simulink model "cascaded_5_lvl"  (R2023a)
settings: Solver=ode4  StartTime=0.0  StopTime=0.1  FixedStep=1e-5  RelTol=1e-3  EnableMultiTasking=on
libraries: spsIGBTDiodeLib x24, simulink x12, spsDCVoltageSourceLib x6, spsSeriesRLCBranchLib x3, spsGroundLib x2, spsThreePhaseVIMeasurementLib x1, spspowerguiLib x1
settings Model: Creator=Rini Roni  LastModifiedBy=dhana
settings SolverCC: AlgebraicLoopSolver=TrustRegion
settings DataIOCC: LimitDataPoints=on  SaveFormat=Array  ReturnWorkspaceOutputs=off
settings OptimizationCC: LifeSpan=inf
settings DebuggingCC: UnderspecifiedInitializationDetection=Classic  MergeDetectMultiDrivingBlocksExec=none  SolverPrmCheckMsg=warning  UnconnectedInputMsg=warning  UnconnectedOutputMsg=warning  UnconnectedLineMsg=warning  StateNameClashWarn=warning  SFUnexpectedBacktrackingDiag=warning  SFNoUnconditionalDefaultTransitionDiag=warning  SFExecutionAtInitializationDiag=none  ArithmeticOperatorsInVariantConditions=warning
settings HardwareCC: ProdBitPerPointer=32  ProdBitPerSizeT=32  ProdBitPerPtrDiffT=32  ProdLargestAtomicFloat=None  ProdIntDivRoundTo=Undefined  ProdEndianess=Unspecified  ProdWordSize=32  ProdHWDeviceType=32-bit Generic
settings ModelReferenceCC: EnableRefExpFcnMdlSchedulingChecks=on  PropagateSignalLabelsOutOfModel=off
settings SFSimCC: SimUseLocalCustomCode=off  CustomCodeUndefinedFunction=UseInterfaceOnly
settings RTWCC: RTWUseLocalCustomCode=off
settings CodeAppCC: StateflowObjectComments=on
settings GRTTargetCC: TargetLangStandard=C89/C90 (ANSI)
settings ConfigComp: CovMetricSettings=dw  CovSaveCumulativeToWorkspaceVar=on  CovSaveSingleToWorkspaceVar=on  CovExternalEMLEnable=off
settings SimscapeCC: SimscapeNormalizeSystem=off

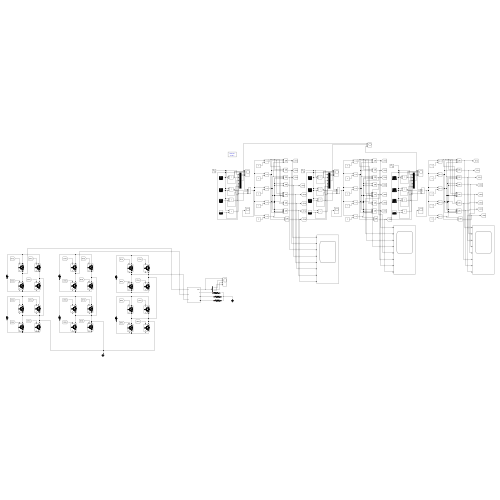
[thumbnail: Simulink's stored preview of the top-level diagram]
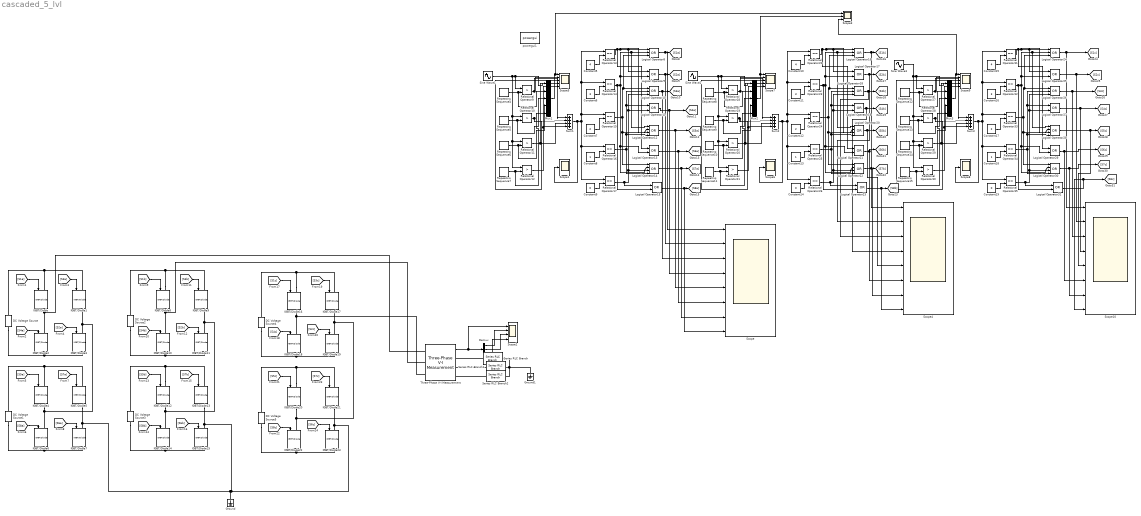
== system cascaded_5_lvl ==
  Constant10 : Constant  Value=4
  Constant11 : Constant  Value=3
  Constant12 : Constant  Value=2
  Constant13 : Constant
  Constant14 : Constant  Value=0
  Constant15 : Constant  Value=4
  Constant16 : Constant  Value=3
  Constant17 : Constant  Value=2
  Constant18 : Constant
  Constant19 : Constant  Value=0
  Constant5 : Constant  Value=4
  Constant6 : Constant  Value=3
  Constant7 : Constant  Value=2
  Constant8 : Constant
  Constant9 : Constant  Value=0
  DC Voltage Source{,1..5} (6 alike) : spsDCVoltageSourceLib/DC Voltage Source  Amplitude=50  Measurements=None
  Demux : Demux  Outputs=3
  Ground : spsGroundLib/Ground  LConnTagsString=a
  Ground1 : spsGroundLib/Ground  LConnTagsString=a
  IGBT/Diode{,1..23} (24 alike) : spsIGBTDiodeLib/IGBT//Diode  Ron=1e-3  Rs=1e5  Cs=inf  Measurements=on
  Logical Operator{8,10,16,18,24,26} (6 alike) : Logic  Operator=OR  Inputs=3  AllPortsSameDT=off  OutDataTypeStr=boolean
  Logical Operator{9,11,13,15,17,19,21,23,25,27,29,31} (12 alike) : Logic  Operator=OR  AllPortsSameDT=off  OutDataTypeStr=boolean
  Logical Operator{12,14,20,22,28,30} (6 alike) : Logic  Operator=OR  Inputs=4  AllPortsSameDT=off  OutDataTypeStr=boolean
  Mux1 : Mux  Inputs=5
  Mux2 : Mux  Inputs=5
  Mux3 : Mux  Inputs=5
  Relational Operator{9..12,18..21,27..30} (12 alike) : RelationalOperator  Operator=>  OutDataTypeStr=boolean  InputSameDT=off
  Relational Operator{13..17,22..26,31..35} (15 alike) : RelationalOperator  Operator===  OutDataTypeStr=boolean  InputSameDT=off
  Repeating Sequence10 : simulink/Sources/Repeating Sequence  rep_seq_t=[0 1 2 ]*[1/5000]  rep_seq_y=[-1 0 -1]
  Repeating Sequence11 : simulink/Sources/Repeating Sequence  rep_seq_t=[0 1 2 ]*[1/5000]  rep_seq_y="[-2  -1 -2]"
  Repeating Sequence12 : simulink/Sources/Repeating Sequence  rep_seq_t=[0 1 2 ]*[1/5000]  rep_seq_y=[1 2 1]
  Repeating Sequence13 : simulink/Sources/Repeating Sequence  rep_seq_t=[0 1 2 ]*[1/5000]  rep_seq_y=[0 1 0]
  Repeating Sequence14 : simulink/Sources/Repeating Sequence  rep_seq_t=[0 1 2 ]*[1/5000]  rep_seq_y=[-1 0 -1]
  Repeating Sequence15 : simulink/Sources/Repeating Sequence  rep_seq_t=[0 1 2 ]*[1/5000]  rep_seq_y="[-2  -1 -2]"
  Repeating Sequence4 : simulink/Sources/Repeating Sequence  rep_seq_t=[0 1 2 ]*[1/5000]  rep_seq_y=[1 2 1]
  Repeating Sequence5 : simulink/Sources/Repeating Sequence  rep_seq_t=[0 1 2 ]*[1/5000]  rep_seq_y=[0 1 0]
  Repeating Sequence6 : simulink/Sources/Repeating Sequence  rep_seq_t=[0 1 2 ]*[1/5000]  rep_seq_y=[-1 0 -1]
  Repeating Sequence7 : simulink/Sources/Repeating Sequence  rep_seq_t=[0 1 2 ]*[1/5000]  rep_seq_y="[-2  -1 -2]"
  Repeating Sequence8 : simulink/Sources/Repeating Sequence  rep_seq_t=[0 1 2 ]*[1/5000]  rep_seq_y=[1 2 1]
  Repeating Sequence9 : simulink/Sources/Repeating Sequence  rep_seq_t=[0 1 2 ]*[1/5000]  rep_seq_y=[0 1 0]
  Scope : Scope  NumInputPorts=8
  Scope1 : Scope
  Scope10 : Scope  NumInputPorts=8
  Scope2 : Scope  NumInputPorts=4
  Scope3 : Scope  NumInputPorts=3
  Scope4 : Scope  NumInputPorts=8
  Scope5 : Scope  NumInputPorts=5
  Scope6 : Scope
  Scope7 : Scope  NumInputPorts=5
  Scope8 : Scope
  Scope9 : Scope  NumInputPorts=5
  Series RLC Branch : spsSeriesRLCBranchLib/Series RLC Branch  LConnTagsString=__new0  RConnTagsString=__new0  BranchType=R  Resistance=500  Inductance=1e-3  SetiL0=off  InitialCurrent=0  Capacitance=1e-6  Setx0=off  InitialVoltage=0  Measurements=Branch voltage
  Series RLC Branch1 : spsSeriesRLCBranchLib/Series RLC Branch  LConnTagsString=__new0  RConnTagsString=__new0  BranchType=R  Resistance=100  Inductance=1e-3  SetiL0=off  InitialCurrent=0  Capacitance=1e-6  Setx0=off  InitialVoltage=0  Measurements=Branch voltage
  Series RLC Branch2 : spsSeriesRLCBranchLib/Series RLC Branch  LConnTagsString=__new0  RConnTagsString=__new0  BranchType=R  Resistance=250  Inductance=1e-3  SetiL0=off  InitialCurrent=0  Capacitance=1e-6  Setx0=off  InitialVoltage=0  Measurements=Branch voltage
  Sine Wave1 : Sin  Amplitude=2  Frequency=2*pi*50  SampleTime=0
  Sine Wave2 : Sin  Amplitude=2  Frequency=2*pi*50  Phase=4*pi/3  SampleTime=0
  Sine Wave3 : Sin  Amplitude=2  Frequency=2*pi*50  Phase=2*pi/3  SampleTime=0
  Sum1 : Sum  Inputs=|++++
  Sum2 : Sum  Inputs=|++++
  Sum3 : Sum  Inputs=|++++
  Three-Phase V-I Measurement : spsThreePhaseVIMeasurementLib/Three-Phase V-I Measurement  VoltageMeasurement=phase-to-ground  SetLabelV=off  LabelV=Vabc  Vpu=off  VpuLL=off  CurrentMeasurement=no  SetLabelI=off  LabelI=Iabc  Ipu=off  Pbase=100e6  Vbase=500e3  OutputType=Complex  PhasorSimulation=off  PSBequivalent=0
  powergui1 : spspowerguiLib/powergui  Priority=1  SimulationMode=Discrete  SampleTime=1e-5  frequency=60  Iterations=50  frequencyindice=0  Pbase=100e6  ErrMax=1e-4  UnitsV=kV  UnitsW=MW  buscounter=0  FunctionMessages=off  echomessages=off  EnableUseOfTLC=off  CurrentSourceSwitches=off  DisableSnubberDevices=off  DisableRonSwitches=off  DisableVfSwitches=off  DisplayEquations=off  AutomaticDiscreteSolvers=off  SolverType=Tustin  Interpol=off  ExternalGateDelay=off  methode=off  Ts=0  x0status=blocks  SPID=off  SwTol=0  HookPort=off  NonlinearTolerance=1e-4  nMaxIteration=100  ContinueOnMaxIteration=off  RestoreLinks=warning  ResistiveCurrentMeasurement=off  Frange=[0:2:500]  Ylog=off  Xlog=on  ShowGrid=off  save=off  variable=ZData  structure=ScopeData  ZoomFFT=off  StartTime=0.02  cycles=1  DisplayStyle=1  fundamental=50  FreqAxis=off  MaxFrequency=1000  frequencyindicesteady=1  RmsSteady=1  display=off
  wires:
  [S1a] -> IGBT/Diode/1
  [S4a] -> IGBT/Diode2/1
  [S3a] -> IGBT/Diode1/1
  [S2a] -> IGBT/Diode3/1
  [S5a] -> IGBT/Diode4/1
  [S8a] -> IGBT/Diode6/1
  [S7a] -> IGBT/Diode5/1
  [S6a] -> IGBT/Diode7/1
  [S1b] -> IGBT/Diode8/1
  [S6b] -> IGBT/Diode15/1
  [S7b] -> IGBT/Diode13/1
  [S8b] -> IGBT/Diode14/1
  [S2b] -> IGBT/Diode11/1
  [S3b] -> IGBT/Diode9/1
  [S4b] -> IGBT/Diode10/1
  [S5b] -> IGBT/Diode12/1
  [S1c] -> IGBT/Diode16/1
  [S6c] -> IGBT/Diode23/1
  [S7c] -> IGBT/Diode21/1
  [S8c] -> IGBT/Diode22/1
  [S2c] -> IGBT/Diode19/1
  [S3c] -> IGBT/Diode17/1
  [S4c] -> IGBT/Diode18/1
  [S5c] -> IGBT/Diode20/1
  Demux/1 -> Scope2/2
  Demux/2 -> Scope2/3
  Demux/3 -> Scope2/4
  Three-Phase V-I Measurement/1 -> Scope2/1, Demux/1
  Relational Operator9/1 -> Sum1/1, Scope5/2
  Relational Operator11/1 -> Sum1/3, Scope5/4
  Constant8/1 -> Relational Operator16/2
  Relational Operator10/1 -> Sum1/2, Scope5/3
  Constant7/1 -> Relational Operator15/2
  Constant5/1 -> Relational Operator13/2
  Repeating Sequence4/1 -> Mux1/2, Relational Operator9/2
  Constant6/1 -> Relational Operator14/2
  Constant9/1 -> Relational Operator17/2
  Repeating Sequence7/1 -> Mux1/5, Relational Operator12/2
  Logical Operator13/1 -> Scope/6, [S6a]
  Sum1/1 -> Scope1/1, Relational Operator15/1, Relational Operator14/1, Relational Operator13/1, Relational Operator17/1, Relational Operator16/1
  Relational Operator13/1 -> Logical Operator13/1, Logical Operator12/3, Logical Operator9/1, Logical Operator8/1
  Relational Operator16/1 -> Logical Operator12/4, Logical Operator11/1, Logical Operator10/2, Logical Operator14/4
  Relational Operator14/1 -> Logical Operator15/2, Logical Operator12/1, Logical Operator8/2, Logical Operator9/2, Logical Operator13/2, Logical Operator14/3
  Repeating Sequence6/1 -> Mux1/4, Relational Operator11/2
  Relational Operator15/1 -> Logical Operator14/1, Logical Operator12/2, Logical Operator10/1, Logical Operator8/3
  Logical Operator10/1 -> Scope/3, [S3a]
  Mux1/1 -> Scope3/1, Scope5/1
  Relational Operator12/1 -> Sum1/4, Scope5/5
  Relational Operator17/1 -> Logical Operator15/1, Logical Operator14/2, Logical Operator11/2, Logical Operator10/3
  Repeating Sequence5/1 -> Mux1/3, Relational Operator10/2
  Logical Operator8/1 -> Scope/1, [S1a]
  Logical Operator12/1 -> Scope/5, [S5a]
  Logical Operator9/1 -> Scope/2, [S2a]
  Logical Operator15/1 -> Scope/8, [S8a]
  Sine Wave1/1 -> Mux1/1, Relational Operator9/1, Relational Operator12/1, Relational Operator11/1, Relational Operator10/1
  Relational Operator18/1 -> Sum2/1, Scope7/2
  Relational Operator20/1 -> Sum2/3, Scope7/4
  Constant13/1 -> Relational Operator25/2
  Relational Operator19/1 -> Sum2/2, Scope7/3
  Constant12/1 -> Relational Operator24/2
  Constant10/1 -> Relational Operator22/2
  Repeating Sequence8/1 -> Mux2/2, Relational Operator18/2
  Constant11/1 -> Relational Operator23/2
  Constant14/1 -> Relational Operator26/2
  Repeating Sequence11/1 -> Mux2/5, Relational Operator21/2
  Logical Operator21/1 -> [S6b], Scope4/6
  Sum2/1 -> Scope6/1, Relational Operator24/1, Relational Operator23/1, Relational Operator22/1, Relational Operator26/1, Relational Operator25/1
  Relational Operator22/1 -> Logical Operator21/1, Logical Operator20/3, Logical Operator17/1, Logical Operator16/1
  Relational Operator25/1 -> Logical Operator20/4, Logical Operator19/1, Logical Operator18/2, Logical Operator22/4
  Relational Operator23/1 -> Logical Operator23/2, Logical Operator20/1, Logical Operator16/2, Logical Operator17/2, Logical Operator21/2, Logical Operator22/3
  Repeating Sequence10/1 -> Mux2/4, Relational Operator20/2
  Relational Operator24/1 -> Logical Operator22/1, Logical Operator20/2, Logical Operator18/1, Logical Operator16/3
  Logical Operator22/1 -> Scope4/7, [S7b]
  Mux2/1 -> Scope3/2, Scope7/1
  Relational Operator21/1 -> Sum2/4, Scope7/5
  Relational Operator26/1 -> Logical Operator23/1, Logical Operator22/2, Logical Operator19/2, Logical Operator18/3
  Repeating Sequence9/1 -> Mux2/3, Relational Operator19/2
  Logical Operator16/1 -> Scope4/1, [S1b]
  Logical Operator20/1 -> Scope4/5, [S5b]
  Logical Operator17/1 -> Scope4/2, [S2b]
  Logical Operator23/1 -> Scope4/8, [S8b]
  Sine Wave2/1 -> Mux2/1, Relational Operator18/1, Relational Operator21/1, Relational Operator20/1, Relational Operator19/1
  Logical Operator19/1 -> Scope4/4, [S4b]
  Relational Operator27/1 -> Sum3/1, Scope9/2
  Relational Operator29/1 -> Sum3/3, Scope9/4
  Constant18/1 -> Relational Operator34/2
  Relational Operator28/1 -> Sum3/2, Scope9/3
  Constant17/1 -> Relational Operator33/2
  Constant15/1 -> Relational Operator31/2
  Repeating Sequence12/1 -> Mux3/2, Relational Operator27/2
  Constant16/1 -> Relational Operator32/2
  Constant19/1 -> Relational Operator35/2
  Repeating Sequence15/1 -> Mux3/5, Relational Operator30/2
  Logical Operator29/1 -> Scope10/6, [S6c]
  Sum3/1 -> Scope8/1, Relational Operator33/1, Relational Operator32/1, Relational Operator31/1, Relational Operator35/1, Relational Operator34/1
  Relational Operator31/1 -> Logical Operator29/1, Logical Operator28/3, Logical Operator25/1, Logical Operator24/1
  Relational Operator34/1 -> Logical Operator28/4, Logical Operator27/1, Logical Operator26/2, Logical Operator30/4
  Relational Operator32/1 -> Logical Operator31/2, Logical Operator28/1, Logical Operator24/2, Logical Operator25/2, Logical Operator29/2, Logical Operator30/3
  Repeating Sequence14/1 -> Mux3/4, Relational Operator29/2
  Relational Operator33/1 -> Logical Operator30/1, Logical Operator28/2, Logical Operator26/1, Logical Operator24/3
  Logical Operator30/1 -> Scope10/7, [S7c]
  Logical Operator26/1 -> Scope10/3, [S3c]
  Mux3/1 -> Scope3/3, Scope9/1
  Relational Operator30/1 -> Sum3/4, Scope9/5
  Relational Operator35/1 -> Logical Operator31/1, Logical Operator30/2, Logical Operator27/2, Logical Operator26/3
  Repeating Sequence13/1 -> Mux3/3, Relational Operator28/2
  Logical Operator24/1 -> Scope10/1, [S1c]
  Logical Operator28/1 -> Scope10/5, [S5c]
  Logical Operator25/1 -> Scope10/2, [S2c]
  Logical Operator31/1 -> [S8c], Scope10/8
  Sine Wave3/1 -> Mux3/1, Relational Operator27/1, Relational Operator30/1, Relational Operator29/1, Relational Operator28/1
  Logical Operator27/1 -> [S4c], Scope10/4
  Logical Operator11/1 -> Scope/4, [S4a]
  Logical Operator14/1 -> Scope/7, [S7a]
  Logical Operator18/1 -> Scope4/3, [S3b]
  connections:
  DC Voltage Source/RConn1 -- IGBT/Diode1/LConn1 -- IGBT/Diode/LConn1
  DC Voltage Source/LConn1 -- IGBT/Diode3/RConn1 -- IGBT/Diode2/RConn1
  DC Voltage Source1/RConn1 -- IGBT/Diode5/LConn1 -- IGBT/Diode4/LConn1
  DC Voltage Source1/LConn1 -- IGBT/Diode6/RConn1 -- IGBT/Diode7/RConn1
  IGBT/Diode3/LConn1 -- IGBT/Diode4/RConn1 -- IGBT/Diode6/LConn1 -- IGBT/Diode1/RConn1
  IGBT/Diode21/RConn1 -- IGBT/Diode7/LConn1 -- IGBT/Diode5/RConn1 -- Ground/LConn1 -- IGBT/Diode13/RConn1 -- IGBT/Diode15/LConn1 -- IGBT/Diode23/LConn1
  IGBT/Diode2/LConn1 -- Three-Phase V-I Measurement/LConn1 -- IGBT/Diode/RConn1
  IGBT/Diode8/LConn1 -- DC Voltage Source2/RConn1 -- IGBT/Diode9/LConn1
  IGBT/Diode12/LConn1 -- DC Voltage Source3/RConn1 -- IGBT/Diode13/LConn1
  IGBT/Diode10/RConn1 -- DC Voltage Source2/LConn1 -- IGBT/Diode11/RConn1
  IGBT/Diode15/RConn1 -- DC Voltage Source3/LConn1 -- IGBT/Diode14/RConn1
  IGBT/Diode11/LConn1 -- IGBT/Diode14/LConn1 -- IGBT/Diode12/RConn1 -- IGBT/Diode9/RConn1
  IGBT/Diode10/LConn1 -- Three-Phase V-I Measurement/LConn2 -- IGBT/Diode8/RConn1
  IGBT/Diode16/LConn1 -- DC Voltage Source4/RConn1 -- IGBT/Diode17/LConn1
  IGBT/Diode20/LConn1 -- DC Voltage Source5/RConn1 -- IGBT/Diode21/LConn1
  IGBT/Diode18/RConn1 -- DC Voltage Source4/LConn1 -- IGBT/Diode19/RConn1
  IGBT/Diode23/RConn1 -- DC Voltage Source5/LConn1 -- IGBT/Diode22/RConn1
  IGBT/Diode19/LConn1 -- IGBT/Diode20/RConn1 -- IGBT/Diode22/LConn1 -- IGBT/Diode17/RConn1
  IGBT/Diode18/LConn1 -- Three-Phase V-I Measurement/LConn3 -- IGBT/Diode16/RConn1
  Series RLC Branch/LConn1 -- Three-Phase V-I Measurement/RConn1
  Series RLC Branch1/LConn1 -- Three-Phase V-I Measurement/RConn2
  Series RLC Branch2/LConn1 -- Three-Phase V-I Measurement/RConn3
  Series RLC Branch/RConn1 -- Ground1/LConn1 -- Series RLC Branch2/RConn1 -- Series RLC Branch1/RConn1
